simulink model "open_loop"  (R2023b)
settings: Solver=FixedStepAuto  StartTime=0.0  StopTime=inf  RelTol=1e-3  EnableMultiTasking=on
libraries: mbedblockslib x5, stm_qeplib x1
settings Model: ExtModeTrigDuration=10  Creator=miche  LastModifiedBy=miche
settings OptimizationCC: EnhancedBackFolding=on  PassReuseOutputArgsAs=Individual arguments  ZeroExternalMemoryAtStartup=off  ZeroInternalMemoryAtStartup=off  MaxStackSize=64  OptimizeBlockOrder=speed  DifferentSizesBufferReuse=on  OptimizationCustomize=off  EfficientTunableParamExpr=on
settings DebuggingCC: ParameterTunabilityLossMsg=error
settings HardwareCC: ProdBitPerPointer=32  ProdBitPerSizeT=32  ProdBitPerPtrDiffT=32  ProdLargestAtomicInteger=Long  ProdLargestAtomicFloat=Double  ProdWordSize=32  ProdLongLongMode=on  ProdHWDeviceType=ARM Compatible->ARM Cortex
settings SFSimCC: MATLABDynamicMemAlloc=off
settings RTWCC: Description=Embedded Coder  SystemTargetFile=ert.tlc  HardwareBoard=STM32 Nucleo F401RE  TemplateMakefile=ert_default_tmf  Toolchain=GNU Tools for ARM Embedded Processors
settings CodeAppCC: ForceParamTrailComments=on  IgnoreCustomStorageClasses=off  OperatorAnnotations=on  SimulinkDataObjDesc=on  SFDataObjDesc=on  InsertBlockDesc=on
settings ERTTargetCC: ExtModeTransport=3  ExtModeStaticAlloc=on  ExtModeStaticAllocSize=2000  ExtModeMexFile=ext_xcp  ExtModeIntrfLevel=Level2 - Open

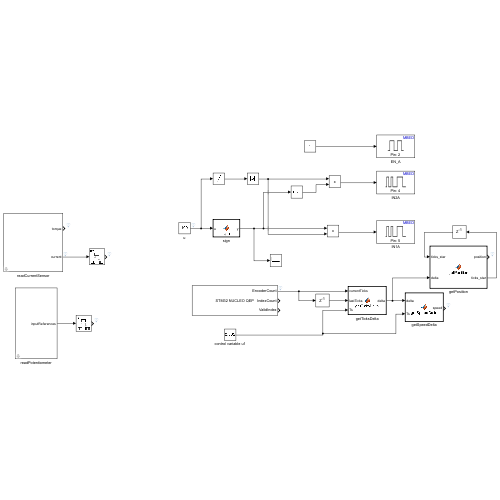
[thumbnail: Simulink's stored preview of the top-level diagram]
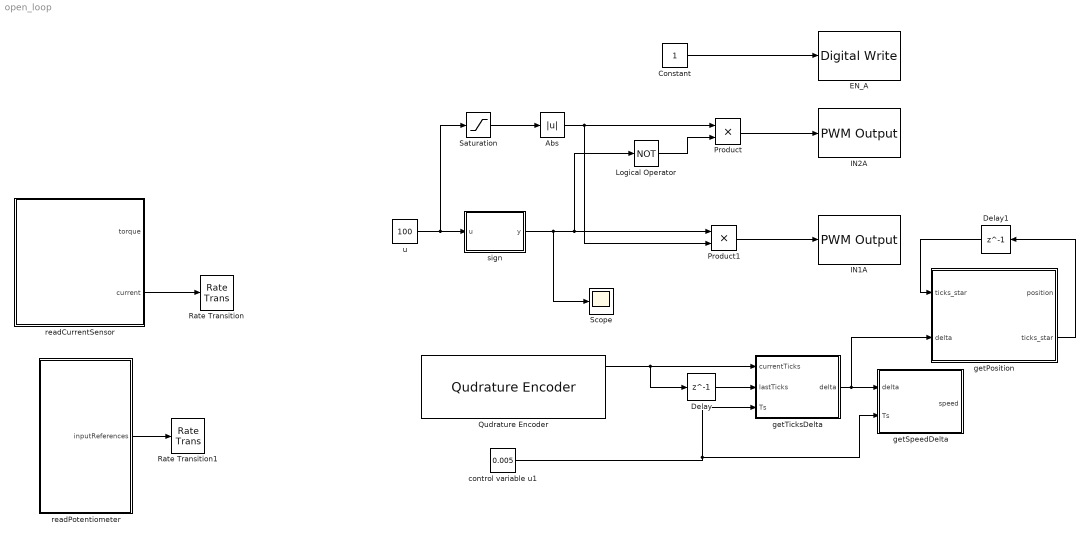
== system open_loop ==
  Abs : Abs  SaturateOnIntegerOverflow=off
  Constant : Constant
  Delay : Delay  DelayLength=1  InitialCondition=0
  Delay1 : Delay  DelayLength=1  InitialCondition=0
  EN_A : mbedblockslib/Digital Write  Pin=2  Direction=output
      settings: LibrarySourceBlock=stmnucleorootlib/Common/Digital Write
  IN1A : mbedblockslib/PWM Output  Pin=5  EnableInputFrequency=off  InitialFrequency=2000  InitialDutyCycle=50  NotificationType=None
      settings: LibrarySourceBlock=stmnucleorootlib/Common/PWM Output
  IN2A : mbedblockslib/PWM Output  Pin=4  EnableInputFrequency=off  InitialFrequency=2000  InitialDutyCycle=50  NotificationType=None
      settings: LibrarySourceBlock=stmnucleorootlib/Common/PWM Output
  Logical Operator : Logic  Operator=NOT  AllPortsSameDT=off  OutDataTypeStr=boolean
  Product : Product
  Product1 : Product
  Qudrature Encoder : stm_qeplib/Qudrature Encoder  SampleTime=0.005
  Rate Transition : RateTransition
  Rate Transition1 : RateTransition
  Saturation : Saturate  UpperLimit=100  LowerLimit=-100
  Scope : Scope
  control variable u1 : Constant  Value=0.005
  getPosition : MATLAB Function  TreatAsAtomicUnit=on
  getSpeedDelta : MATLAB Function  TreatAsAtomicUnit=on
  getTicksDelta : MATLAB Function  TreatAsAtomicUnit=on
  readCurrentSensor : Subsystem  mask{alpha=0.9}
  readPotentiometer : Subsystem  mask{alpha=0.9}
  sign : MATLAB Function  TreatAsAtomicUnit=on
  u : Constant  Value=100
  wires:
  Constant/1 -> EN_A/1
  Product/1 -> IN2A/1
  u/1 -> sign/1(u), Saturation/1
  Saturation/1 -> Abs/1
  Abs/1 -> Product1/2, Product/1
  sign/1(y) -> Scope/1, Product1/1, Logical Operator/1
  Logical Operator/1 -> Product/2
  Product1/1 -> IN1A/1
  control variable u1/1 -> getSpeedDelta/2(Ts), getTicksDelta/3(Ts)
  getTicksDelta/1(delta) -> getPosition/2(delta), getSpeedDelta/1(delta)
  Delay/1 -> getTicksDelta/2(lastTicks)
  Qudrature Encoder/1 -> Delay/1, getTicksDelta/1(currentTicks)
  getPosition/2(ticks_star) -> Delay1/1
  Delay1/1 -> getPosition/1("ticks_star ")
  readCurrentSensor/2(current) -> Rate Transition/1
  readPotentiometer/1(inputReferences) -> Rate Transition1/1

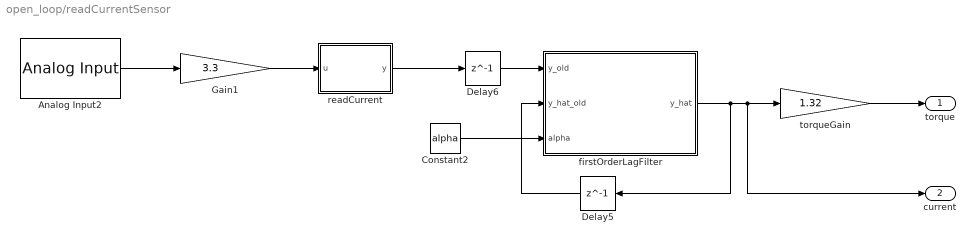
== system open_loop/readCurrentSensor ==
  Analog Input2 : mbedblockslib/Analog Input  Pin=A5  ReadResultsOnly=off  ConversionTriggerSource=Software  ExternalTriggerType=uint32( 0 )  OutputDataType=double  EnableConversionCompleteNotify=off  EnableOuputStatus=off  SampleTime=0.005/20
      settings: LibrarySourceBlock=stmnucleorootlib/Common/Analog Input
  Constant2 : Constant  Value=alpha
  Delay5 : Delay  DelayLength=1  InitialCondition=0
  Delay6 : Delay  DelayLength=1  InitialCondition=0
  Gain1 : Gain  Gain=3.3
  firstOrderLagFilter : MATLAB Function  TreatAsAtomicUnit=on
  readCurrent : MATLAB Function  TreatAsAtomicUnit=on
  torqueGain : Gain  Gain=1.32
  torque : Outport
  current : Outport  Port=2
  wires:
  Constant2/1 -> firstOrderLagFilter/3(alpha)
  firstOrderLagFilter/1(y_hat) -> current/1, torqueGain/1, Delay5/1
  torqueGain/1 -> torque/1
  Gain1/1 -> readCurrent/1(u)
  Analog Input2/1 -> Gain1/1
  readCurrent/1(y) -> Delay6/1
  Delay5/1 -> firstOrderLagFilter/2(y_hat_old)
  Delay6/1 -> firstOrderLagFilter/1(y_old)

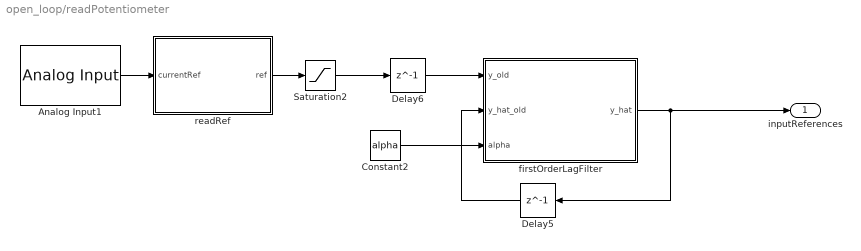
== system open_loop/readPotentiometer ==
  Analog Input1 : mbedblockslib/Analog Input  Pin=A4  ReadResultsOnly=off  ConversionTriggerSource=Software  ExternalTriggerType=uint32( 0 )  OutputDataType=double  EnableConversionCompleteNotify=off  EnableOuputStatus=off  SampleTime=0.005/20
      settings: LibrarySourceBlock=stmnucleorootlib/Common/Analog Input
  Constant2 : Constant  Value=alpha
  Delay5 : Delay  DelayLength=1  InitialCondition=0
  Delay6 : Delay  DelayLength=1  InitialCondition=0
  Saturation2 : Saturate  UpperLimit=0.2  LowerLimit=0
  firstOrderLagFilter : MATLAB Function  TreatAsAtomicUnit=on
  readRef : MATLAB Function  TreatAsAtomicUnit=on
  inputReferences : Outport
  wires:
  Saturation2/1 -> Delay6/1
  Delay6/1 -> firstOrderLagFilter/1(y_old)
  readRef/1(ref) -> Saturation2/1
  Constant2/1 -> firstOrderLagFilter/3(alpha)
  Delay5/1 -> firstOrderLagFilter/2(y_hat_old)
  firstOrderLagFilter/1(y_hat) -> inputReferences/1, Delay5/1
  Analog Input1/1 -> readRef/1(currentRef)

== matlab function open_loop/getTicksDelta ==
  data: currentTicks input; delta output; lastTicks input; Ts input
function delta = getTicksDelta(currentTicks,lastTicks, Ts)

currentTicks=double(currentTicks);
lastTicks=double(lastTicks);

if abs(currentTicks -lastTicks) <= ceil(12600*Ts)
    delta= currentTicks - lastTicks;
else
    if lastTicks > currentTicks
        delta= currentTicks + 2^16 -1 - lastTicks;
    else
        delta= currentTicks - 2^16 +1 - lastTicks;
    end
end

end

== matlab function open_loop/sign ==
  data: u input; y output
function y = sign(u)
if u >0
    y=1;
else
   y=0;
end

== matlab function open_loop/getSpeedDelta ==
  data: delta input; speed output; Ts input
function speed=getSpeedDelta(delta,Ts)
speed=delta * 60/ (8400*Ts);
end

== matlab function open_loop/getPosition ==
  data: ticks_star input; delta input; position output; ticks_star output
function [position,ticks_star] = getPosition(ticks_star, delta)
    ticks_star=double(ticks_star + delta);
    completeTheta=2*pi*ticks_star/(8400);
    position=sign(completeTheta)*mod(abs(completeTheta), 2*pi)
end

== matlab function open_loop/readCurrentSensor/firstOrderLagFilter ==
  data: y_old input; y_hat output; y_hat_old input; alpha input
function y_hat = firstOrderLagFilter(y_old, y_hat_old, alpha)
    y_hat= (alpha *y_hat_old) + ((1-alpha)* y_old)
end

== matlab function open_loop/readCurrentSensor/readCurrent ==
  data: u input; y output
function y = readCurrent(u)


y=(u-2.5-0.105)/0.185

== matlab function open_loop/readPotentiometer/firstOrderLagFilter ==
  data: y_old input; y_hat output; y_hat_old input; alpha input
function y_hat = firstOrderLagFilter(y_old, y_hat_old, alpha)
    y_hat= (alpha *y_hat_old) + ((1-alpha)* y_old)
end

== matlab function open_loop/readPotentiometer/readRef ==
  data: currentRef input; ref output
function ref= getRef(currentRef) 
    
    ref = currentRef * 0.2
end
